simulink model "System_20220515"  (R2020b)
settings: Solver=ode4  StartTime=0.0  StopTime=inf  FixedStep=Ts  RelTol=1e-3  EnableMultiTasking=on
PreLoadFcn:
  | simulation_vars
PostLoadFcn:
  | simulation_vars
InitFcn:
  | simulation_vars
StartFcn:
  | simulation_vars
values from neighbouring files (symbols this model uses):
  ang_variance = 0.001*60    (= 0.06)    [simulation_vars.m]
  bus_va_seed = abs(round(1000*randn(73,1)))    [simulation_vars.m]
  bus_vm_seed = abs(round(1000*randn(73,1)))    [simulation_vars.m]
  event_time_end = event_time_start + 5/60    (= 10000.0833333)    [simulation_vars.m]
  event_time_start = 10000    [simulation_vars.m]
  line_iang0_seed = abs(round(1000*randn(104,1)))    [simulation_vars.m]
  line_iang1_seed = abs(round(1000*randn(104,1)))    [simulation_vars.m]
  line_imag0_seed = abs(round(1000*randn(104,1)))    [simulation_vars.m]
  line_imag1_seed = abs(round(1000*randn(104,1)))    [simulation_vars.m]
  mag_variance = 0.0005    [simulation_vars.m]
  spoof_lower_limit = -pi()/9    [simulation_vars.m]
  spoof_upper_limit = pi()/9    [simulation_vars.m]
  Ts = 0.001    [simulation_vars.m]
  xf_iang0_seed = abs(round(1000*randn(16,1)))    [simulation_vars.m]
  xf_iang1_seed = abs(round(1000*randn(16,1)))    [simulation_vars.m]
  xf_imag0_seed = abs(round(1000*randn(16,1)))    [simulation_vars.m]
  xf_imag1_seed = abs(round(1000*randn(16,1)))    [simulation_vars.m]
undefined symbols (not defined in the file or in its folder): en_spoofing_attack
libraries: rtlab x210, simulink x21, opal_lib x1, rtlab_phasor x1, rtio_spectracom x1
(part 2 of 4)

== system System_20220515/sm_master/PMU202_signals ==
  In1 : Inport
  Demux : Demux  Outputs=8
  PMU202_I1a : rtlab/OpOutput  identifier_use=PMU202_I1a  identifier_hide=PMU202_I1a  nb_parents_identifier=0
      settings: SourceProductName=RT-LAB
  PMU202_I1m : rtlab/OpOutput  identifier_use=PMU202_I1m  identifier_hide=PMU202_I1m  nb_parents_identifier=0
      settings: SourceProductName=RT-LAB
  PMU202_I2a : rtlab/OpOutput  identifier_use=PMU202_I2a  identifier_hide=PMU202_I2a  nb_parents_identifier=0
      settings: SourceProductName=RT-LAB
  PMU202_I2m : rtlab/OpOutput  identifier_use=PMU202_I2m  identifier_hide=PMU202_I2m  nb_parents_identifier=0
      settings: SourceProductName=RT-LAB
  PMU202_I3a : rtlab/OpOutput  identifier_use=PMU202_I3a  identifier_hide=PMU202_I3a  nb_parents_identifier=0
      settings: SourceProductName=RT-LAB
  PMU202_I3m : rtlab/OpOutput  identifier_use=PMU202_I3m  identifier_hide=PMU202_I3m  nb_parents_identifier=0
      settings: SourceProductName=RT-LAB
  PMU202_Va : rtlab/OpOutput  identifier_use=PMU202_Va  identifier_hide=PMU202_Va  nb_parents_identifier=0
      settings: SourceProductName=RT-LAB
  PMU202_Vm : rtlab/OpOutput  identifier_use=PMU202_Vm  identifier_hide=PMU202_Vm  nb_parents_identifier=0
      settings: SourceProductName=RT-LAB
  Spoofing attack : Subsystem
  Out1 : Outport  VectorParamsAs1DForOutWhenUnconnected=off
  wires:
  Demux/3 -> PMU202_I1m/1
  Demux/1 -> PMU202_Vm/1
  Demux/6 -> PMU202_I2a/1
  Demux/2 -> PMU202_Va/1
  Demux/4 -> PMU202_I1a/1
  Demux/5 -> PMU202_I2m/1
  In1/1 -> Spoofing attack/1(Input)
  Demux/7 -> PMU202_I3m/1
  Demux/8 -> PMU202_I3a/1
  Spoofing attack/1(Output) -> Out1/1, Demux/1

== system System_20220515/sm_master/PMU203_signals ==
  In1 : Inport
  Demux : Demux  Outputs=10
  PMU203_I1a : rtlab/OpOutput  identifier_use=PMU203_I1a  identifier_hide=PMU203_I1a  nb_parents_identifier=0
      settings: SourceProductName=RT-LAB
  PMU203_I1m : rtlab/OpOutput  identifier_use=PMU203_I1m  identifier_hide=PMU203_I1m  nb_parents_identifier=0
      settings: SourceProductName=RT-LAB
  PMU203_I2a : rtlab/OpOutput  identifier_use=PMU203_I2a  identifier_hide=PMU203_I2a  nb_parents_identifier=0
      settings: SourceProductName=RT-LAB
  PMU203_I2m : rtlab/OpOutput  identifier_use=PMU203_I2m  identifier_hide=PMU203_I2m  nb_parents_identifier=0
      settings: SourceProductName=RT-LAB
  PMU203_I3a : rtlab/OpOutput  identifier_use=PMU203_I3a  identifier_hide=PMU203_I3a  nb_parents_identifier=0
      settings: SourceProductName=RT-LAB
  PMU203_I3m : rtlab/OpOutput  identifier_use=PMU203_I3m  identifier_hide=PMU203_I3m  nb_parents_identifier=0
      settings: SourceProductName=RT-LAB
  PMU203_I4a : rtlab/OpOutput  identifier_use=PMU203_I4a  identifier_hide=PMU203_I4a  nb_parents_identifier=0
      settings: SourceProductName=RT-LAB
  PMU203_I4m : rtlab/OpOutput  identifier_use=PMU203_I4m  identifier_hide=PMU203_I4m  nb_parents_identifier=0
      settings: SourceProductName=RT-LAB
  PMU203_Va : rtlab/OpOutput  identifier_use=PMU203_Va  identifier_hide=PMU203_Va  nb_parents_identifier=0
      settings: SourceProductName=RT-LAB
  PMU203_Vm : rtlab/OpOutput  identifier_use=PMU203_Vm  identifier_hide=PMU203_Vm  nb_parents_identifier=0
      settings: SourceProductName=RT-LAB
  Spoofing attack : Subsystem
  Out1 : Outport  VectorParamsAs1DForOutWhenUnconnected=off
  wires:
  Demux/10 -> PMU203_I4a/1
  Demux/3 -> PMU203_I1m/1
  Demux/1 -> PMU203_Vm/1
  Demux/6 -> PMU203_I2a/1
  Demux/8 -> PMU203_I3a/1
  Demux/2 -> PMU203_Va/1
  Demux/7 -> PMU203_I3m/1
  Demux/4 -> PMU203_I1a/1
  Demux/5 -> PMU203_I2m/1
  Demux/9 -> PMU203_I4m/1
  In1/1 -> Spoofing attack/1(Input)
  Spoofing attack/1(Output) -> Demux/1, Out1/1

== system System_20220515/sm_master/PMU207_signals ==
  In1 : Inport
  Demux : Demux
  PMU207_I1a : rtlab/OpOutput  identifier_use=PMU207_I1a  identifier_hide=PMU207_I1a  nb_parents_identifier=0
      settings: SourceProductName=RT-LAB
  PMU207_I1m : rtlab/OpOutput  identifier_use=PMU207_I1m  identifier_hide=PMU207_I1m  nb_parents_identifier=0
      settings: SourceProductName=RT-LAB
  PMU207_Va : rtlab/OpOutput  identifier_use=PMU207_Va  identifier_hide=PMU207_Va  nb_parents_identifier=0
      settings: SourceProductName=RT-LAB
  PMU207_Vm : rtlab/OpOutput  identifier_use=PMU207_Vm  identifier_hide=PMU207_Vm  nb_parents_identifier=0
      settings: SourceProductName=RT-LAB
  Spoofing attack : Subsystem
  Out1 : Outport  VectorParamsAs1DForOutWhenUnconnected=off
  wires:
  Demux/1 -> PMU207_Vm/1
  Demux/2 -> PMU207_Va/1
  Demux/4 -> PMU207_I1a/1
  Demux/3 -> PMU207_I1m/1
  In1/1 -> Spoofing attack/1(Input)
  Spoofing attack/1(Output) -> Out1/1, Demux/1

== system System_20220515/sm_master/PMU210_signals ==
  Input : Inport
  Demux : Demux  Outputs=12
  PMU210_I1a : rtlab/OpOutput  identifier_use=PMU210_I1a  identifier_hide=PMU210_I1a  nb_parents_identifier=0
      settings: SourceProductName=RT-LAB
  PMU210_I1m : rtlab/OpOutput  identifier_use=PMU210_I1m  identifier_hide=PMU210_I1m  nb_parents_identifier=0
      settings: SourceProductName=RT-LAB
  PMU210_I2a : rtlab/OpOutput  identifier_use=PMU210_I2a  identifier_hide=PMU210_I2a  nb_parents_identifier=0
      settings: SourceProductName=RT-LAB
  PMU210_I2m : rtlab/OpOutput  identifier_use=PMU210_I2m  identifier_hide=PMU210_I2m  nb_parents_identifier=0
      settings: SourceProductName=RT-LAB
  PMU210_I3a : rtlab/OpOutput  identifier_use=PMU210_I3a  identifier_hide=PMU210_I3a  nb_parents_identifier=0
      settings: SourceProductName=RT-LAB
  PMU210_I3m : rtlab/OpOutput  identifier_use=PMU210_I3m  identifier_hide=PMU210_I3m  nb_parents_identifier=0
      settings: SourceProductName=RT-LAB
  PMU210_I4a : rtlab/OpOutput  identifier_use=PMU210_I4a  identifier_hide=PMU210_I4a  nb_parents_identifier=0
      settings: SourceProductName=RT-LAB
  PMU210_I4m : rtlab/OpOutput  identifier_use=PMU210_I4m  identifier_hide=PMU210_I4m  nb_parents_identifier=0
      settings: SourceProductName=RT-LAB
  PMU210_I5a : rtlab/OpOutput  identifier_use=PMU210_I5a  identifier_hide=PMU210_I5a  nb_parents_identifier=0
      settings: SourceProductName=RT-LAB
  PMU210_I5m : rtlab/OpOutput  identifier_use=PMU210_I5m  identifier_hide=PMU210_I5m  nb_parents_identifier=0
      settings: SourceProductName=RT-LAB
  PMU210_Va : rtlab/OpOutput  identifier_use=PMU210_Va  identifier_hide=PMU210_Va  nb_parents_identifier=0
      settings: SourceProductName=RT-LAB
  PMU210_Vm : rtlab/OpOutput  identifier_use=PMU210_Vm  identifier_hide=PMU210_Vm  nb_parents_identifier=0
      settings: SourceProductName=RT-LAB
  Spoofing attack : Subsystem
  Output : Outport  VectorParamsAs1DForOutWhenUnconnected=off
  wires:
  Demux/1 -> PMU210_Vm/1
  Demux/2 -> PMU210_Va/1
  Demux/3 -> PMU210_I1m/1
  Demux/4 -> PMU210_I1a/1
  Demux/8 -> PMU210_I3a/1
  Demux/9 -> PMU210_I4m/1
  Demux/10 -> PMU210_I4a/1
  Demux/11 -> PMU210_I5m/1
  Demux/12 -> PMU210_I5a/1
  Demux/5 -> PMU210_I2m/1
  Demux/6 -> PMU210_I2a/1
  Demux/7 -> PMU210_I3m/1
  Input/1 -> Spoofing attack/1(Input)
  Spoofing attack/1(Output) -> Output/1, Demux/1

== system System_20220515/sm_master/PMU216_signals ==
  In1 : Inport
  Demux : Demux  Outputs=10
  PMU216_I1a : rtlab/OpOutput  identifier_use=PMU216_I1a  identifier_hide=PMU216_I1a  nb_parents_identifier=0
      settings: SourceProductName=RT-LAB
  PMU216_I1m : rtlab/OpOutput  identifier_use=PMU216_I1m  identifier_hide=PMU216_I1m  nb_parents_identifier=0
      settings: SourceProductName=RT-LAB
  PMU216_I2a : rtlab/OpOutput  identifier_use=PMU216_I2a  identifier_hide=PMU216_I2a  nb_parents_identifier=0
      settings: SourceProductName=RT-LAB
  PMU216_I2m : rtlab/OpOutput  identifier_use=PMU216_I2m  identifier_hide=PMU216_I2m  nb_parents_identifier=0
      settings: SourceProductName=RT-LAB
  PMU216_I3a : rtlab/OpOutput  identifier_use=PMU216_I3a  identifier_hide=PMU216_I3a  nb_parents_identifier=0
      settings: SourceProductName=RT-LAB
  PMU216_I3m : rtlab/OpOutput  identifier_use=PMU216_I3m  identifier_hide=PMU216_I3m  nb_parents_identifier=0
      settings: SourceProductName=RT-LAB
  PMU216_I4a : rtlab/OpOutput  identifier_use=PMU216_I4a  identifier_hide=PMU216_I4a  nb_parents_identifier=0
      settings: SourceProductName=RT-LAB
  PMU216_I4m : rtlab/OpOutput  identifier_use=PMU216_I4m  identifier_hide=PMU216_I4m  nb_parents_identifier=0
      settings: SourceProductName=RT-LAB
  PMU216_Va : rtlab/OpOutput  identifier_use=PMU216_Va  identifier_hide=PMU216_Va  nb_parents_identifier=0
      settings: SourceProductName=RT-LAB
  PMU216_Vm : rtlab/OpOutput  identifier_use=PMU216_Vm  identifier_hide=PMU216_Vm  nb_parents_identifier=0
      settings: SourceProductName=RT-LAB
  Spoofing attack : Subsystem
  Out1 : Outport  VectorParamsAs1DForOutWhenUnconnected=off
  wires:
  Demux/10 -> PMU216_I4a/1
  Demux/3 -> PMU216_I1m/1
  Demux/1 -> PMU216_Vm/1
  Demux/6 -> PMU216_I2a/1
  Demux/8 -> PMU216_I3a/1
  Demux/2 -> PMU216_Va/1
  Demux/7 -> PMU216_I3m/1
  Demux/4 -> PMU216_I1a/1
  Demux/5 -> PMU216_I2m/1
  Demux/9 -> PMU216_I4m/1
  In1/1 -> Spoofing attack/1(Input)
  Spoofing attack/1(Output) -> Demux/1, Out1/1

== system System_20220515/sm_master/PMU221_signals ==
  In1 : Inport
  Demux : Demux  Outputs=12
  PMU221_I1a : rtlab/OpOutput  identifier_use=PMU221_I1a  identifier_hide=PMU221_I1a  nb_parents_identifier=0
      settings: SourceProductName=RT-LAB
  PMU221_I1m : rtlab/OpOutput  identifier_use=PMU221_I1m  identifier_hide=PMU221_I1m  nb_parents_identifier=0
      settings: SourceProductName=RT-LAB
  PMU221_I2a : rtlab/OpOutput  identifier_use=PMU221_I2a  identifier_hide=PMU221_I2a  nb_parents_identifier=0
      settings: SourceProductName=RT-LAB
  PMU221_I2m : rtlab/OpOutput  identifier_use=PMU221_I2m  identifier_hide=PMU221_I2m  nb_parents_identifier=0
      settings: SourceProductName=RT-LAB
  PMU221_I3a : rtlab/OpOutput  identifier_use=PMU221_I3a  identifier_hide=PMU221_I3a  nb_parents_identifier=0
      settings: SourceProductName=RT-LAB
  PMU221_I3m : rtlab/OpOutput  identifier_use=PMU221_I3m  identifier_hide=PMU221_I3m  nb_parents_identifier=0
      settings: SourceProductName=RT-LAB
  PMU221_I4a : rtlab/OpOutput  identifier_use=PMU221_I4a  identifier_hide=PMU221_I4a  nb_parents_identifier=0
      settings: SourceProductName=RT-LAB
  PMU221_I4m : rtlab/OpOutput  identifier_use=PMU221_I4m  identifier_hide=PMU221_I4m  nb_parents_identifier=0
      settings: SourceProductName=RT-LAB
  PMU221_I5a : rtlab/OpOutput  identifier_use=PMU221_I5a  identifier_hide=PMU221_I5a  nb_parents_identifier=0
      settings: SourceProductName=RT-LAB
  PMU221_I5m : rtlab/OpOutput  identifier_use=PMU221_I5m  identifier_hide=PMU221_I5m  nb_parents_identifier=0
      settings: SourceProductName=RT-LAB
  PMU221_Va : rtlab/OpOutput  identifier_use=PMU221_Va  identifier_hide=PMU221_Va  nb_parents_identifier=0
      settings: SourceProductName=RT-LAB
  PMU221_Vm : rtlab/OpOutput  identifier_use=PMU221_Vm  identifier_hide=PMU221_Vm  nb_parents_identifier=0
      settings: SourceProductName=RT-LAB
  Spoofing attack : Subsystem
  Out1 : Outport  VectorParamsAs1DForOutWhenUnconnected=off
  wires:
  Demux/1 -> PMU221_Vm/1
  Demux/2 -> PMU221_Va/1
  Demux/3 -> PMU221_I1m/1
  Demux/4 -> PMU221_I1a/1
  Demux/8 -> PMU221_I3a/1
  Demux/9 -> PMU221_I4m/1
  Demux/10 -> PMU221_I4a/1
  Demux/11 -> PMU221_I5m/1
  Demux/12 -> PMU221_I5a/1
  Demux/5 -> PMU221_I2m/1
  Demux/6 -> PMU221_I2a/1
  Demux/7 -> PMU221_I3m/1
  In1/1 -> Spoofing attack/1(Input)
  Spoofing attack/1(Output) -> Out1/1, Demux/1

== system System_20220515/sm_master/PMU223_signals ==
  Input : Inport
  Demux : Demux  Outputs=12
  PMU223_I1a : rtlab/OpOutput  identifier_use=PMU223_I1a  identifier_hide=PMU223_I1a  nb_parents_identifier=0
      settings: SourceProductName=RT-LAB
  PMU223_I1m : rtlab/OpOutput  identifier_use=PMU223_I1m  identifier_hide=PMU223_I1m  nb_parents_identifier=0
      settings: SourceProductName=RT-LAB
  PMU223_I2a : rtlab/OpOutput  identifier_use=PMU223_I2a  identifier_hide=PMU223_I2a  nb_parents_identifier=0
      settings: SourceProductName=RT-LAB
  PMU223_I2m : rtlab/OpOutput  identifier_use=PMU223_I2m  identifier_hide=PMU223_I2m  nb_parents_identifier=0
      settings: SourceProductName=RT-LAB
  PMU223_I3a : rtlab/OpOutput  identifier_use=PMU223_I3a  identifier_hide=PMU223_I3a  nb_parents_identifier=0
      settings: SourceProductName=RT-LAB
  PMU223_I3m : rtlab/OpOutput  identifier_use=PMU223_I3m  identifier_hide=PMU223_I3m  nb_parents_identifier=0
      settings: SourceProductName=RT-LAB
  PMU223_I4a : rtlab/OpOutput  identifier_use=PMU223_I4a  identifier_hide=PMU223_I4a  nb_parents_identifier=0
      settings: SourceProductName=RT-LAB
  PMU223_I4m : rtlab/OpOutput  identifier_use=PMU223_I4m  identifier_hide=PMU223_I4m  nb_parents_identifier=0
      settings: SourceProductName=RT-LAB
  PMU223_I5a : rtlab/OpOutput  identifier_use=PMU223_I5a  identifier_hide=PMU223_I5a  nb_parents_identifier=0
      settings: SourceProductName=RT-LAB
  PMU223_I5m : rtlab/OpOutput  identifier_use=PMU223_I5m  identifier_hide=PMU223_I5m  nb_parents_identifier=0
      settings: SourceProductName=RT-LAB
  PMU223_Va : rtlab/OpOutput  identifier_use=PMU223_Va  identifier_hide=PMU223_Va  nb_parents_identifier=0
      settings: SourceProductName=RT-LAB
  PMU223_Vm : rtlab/OpOutput  identifier_use=PMU223_Vm  identifier_hide=PMU223_Vm  nb_parents_identifier=0
      settings: SourceProductName=RT-LAB
  Spoofing attack : Subsystem
  Output : Outport  VectorParamsAs1DForOutWhenUnconnected=off
  wires:
  Demux/1 -> PMU223_Vm/1
  Demux/2 -> PMU223_Va/1
  Demux/3 -> PMU223_I1m/1
  Demux/4 -> PMU223_I1a/1
  Demux/8 -> PMU223_I3a/1
  Demux/9 -> PMU223_I4m/1
  Demux/10 -> PMU223_I4a/1
  Demux/11 -> PMU223_I5m/1
  Demux/12 -> PMU223_I5a/1
  Demux/5 -> PMU223_I2m/1
  Demux/6 -> PMU223_I2a/1
  Demux/7 -> PMU223_I3m/1
  Input/1 -> Spoofing attack/1(Input)
  Spoofing attack/1(Output) -> Output/1, Demux/1

== system System_20220515/sm_master/PMU302_signals ==
  In1 : Inport
  Demux : Demux  Outputs=8
  PMU302_I1a : rtlab/OpOutput  identifier_use=PMU302_I1a  identifier_hide=PMU302_I1a  nb_parents_identifier=0
      settings: SourceProductName=RT-LAB
  PMU302_I1m : rtlab/OpOutput  identifier_use=PMU302_I1m  identifier_hide=PMU302_I1m  nb_parents_identifier=0
      settings: SourceProductName=RT-LAB
  PMU302_I2a : rtlab/OpOutput  identifier_use=PMU302_I2a  identifier_hide=PMU302_I2a  nb_parents_identifier=0
      settings: SourceProductName=RT-LAB
  PMU302_I2m : rtlab/OpOutput  identifier_use=PMU302_I2m  identifier_hide=PMU302_I2m  nb_parents_identifier=0
      settings: SourceProductName=RT-LAB
  PMU302_I3a : rtlab/OpOutput  identifier_use=PMU302_I3a  identifier_hide=PMU302_I3a  nb_parents_identifier=0
      settings: SourceProductName=RT-LAB
  PMU302_I3m : rtlab/OpOutput  identifier_use=PMU302_I3m  identifier_hide=PMU302_I3m  nb_parents_identifier=0
      settings: SourceProductName=RT-LAB
  PMU302_Va : rtlab/OpOutput  identifier_use=PMU302_Va  identifier_hide=PMU302_Va  nb_parents_identifier=0
      settings: SourceProductName=RT-LAB
  PMU302_Vm : rtlab/OpOutput  identifier_use=PMU302_Vm  identifier_hide=PMU302_Vm  nb_parents_identifier=0
      settings: SourceProductName=RT-LAB
  Spoofing attack : Subsystem
  Out1 : Outport  VectorParamsAs1DForOutWhenUnconnected=off
  wires:
  In1/1 -> Spoofing attack/1(Input)
  Demux/2 -> PMU302_Va/1
  Demux/1 -> PMU302_Vm/1
  Demux/3 -> PMU302_I1m/1
  Demux/4 -> PMU302_I1a/1
  Demux/5 -> PMU302_I2m/1
  Demux/6 -> PMU302_I2a/1
  Demux/7 -> PMU302_I3m/1
  Demux/8 -> PMU302_I3a/1
  Spoofing attack/1(Output) -> Out1/1, Demux/1

== system System_20220515/sm_master/PMU303_signals ==
  In1 : Inport
  Demux : Demux  Outputs=8
  PMU303_I1a : rtlab/OpOutput  identifier_use=PMU303_I1a  identifier_hide=PMU303_I1a  nb_parents_identifier=0
      settings: SourceProductName=RT-LAB
  PMU303_I1m : rtlab/OpOutput  identifier_use=PMU303_I1m  identifier_hide=PMU303_I1m  nb_parents_identifier=0
      settings: SourceProductName=RT-LAB
  PMU303_I2a : rtlab/OpOutput  identifier_use=PMU303_I2a  identifier_hide=PMU303_I2a  nb_parents_identifier=0
      settings: SourceProductName=RT-LAB
  PMU303_I2m : rtlab/OpOutput  identifier_use=PMU303_I2m  identifier_hide=PMU303_I2m  nb_parents_identifier=0
      settings: SourceProductName=RT-LAB
  PMU303_I3a : rtlab/OpOutput  identifier_use=PMU303_I3a  identifier_hide=PMU303_I3a  nb_parents_identifier=0
      settings: SourceProductName=RT-LAB
  PMU303_I3m : rtlab/OpOutput  identifier_use=PMU303_I3m  identifier_hide=PMU303_I3m  nb_parents_identifier=0
      settings: SourceProductName=RT-LAB
  PMU303_Va : rtlab/OpOutput  identifier_use=PMU303_Va  identifier_hide=PMU303_Va  nb_parents_identifier=0
      settings: SourceProductName=RT-LAB
  PMU303_Vm : rtlab/OpOutput  identifier_use=PMU303_Vm  identifier_hide=PMU303_Vm  nb_parents_identifier=0
      settings: SourceProductName=RT-LAB
  Spoofing attack : Subsystem
  Out1 : Outport  VectorParamsAs1DForOutWhenUnconnected=off
  wires:
  In1/1 -> Spoofing attack/1(Input)
  Demux/1 -> PMU303_Vm/1
  Demux/2 -> PMU303_Va/1
  Demux/3 -> PMU303_I1m/1
  Demux/4 -> PMU303_I1a/1
  Demux/5 -> PMU303_I2m/1
  Demux/6 -> PMU303_I2a/1
  Demux/7 -> PMU303_I3m/1
  Demux/8 -> PMU303_I3a/1
  Spoofing attack/1(Output) -> Out1/1, Demux/1

== system System_20220515/sm_master/PMU307_signals ==
  In1 : Inport
  Demux : Demux
  PMU307_I1a : rtlab/OpOutput  identifier_use=PMU307_I1a  identifier_hide=PMU307_I1a  nb_parents_identifier=0
      settings: SourceProductName=RT-LAB
  PMU307_I1m : rtlab/OpOutput  identifier_use=PMU307_I1m  identifier_hide=PMU307_I1m  nb_parents_identifier=0
      settings: SourceProductName=RT-LAB
  PMU307_Va : rtlab/OpOutput  identifier_use=PMU307_Va  identifier_hide=PMU307_Va  nb_parents_identifier=0
      settings: SourceProductName=RT-LAB
  PMU307_Vm : rtlab/OpOutput  identifier_use=PMU307_Vm  identifier_hide=PMU307_Vm  nb_parents_identifier=0
      settings: SourceProductName=RT-LAB
  Spoofing attack : Subsystem
  Out1 : Outport  VectorParamsAs1DForOutWhenUnconnected=off
  wires:
  In1/1 -> Spoofing attack/1(Input)
  Demux/1 -> PMU307_Vm/1
  Demux/2 -> PMU307_Va/1
  Demux/4 -> PMU307_I1a/1
  Demux/3 -> PMU307_I1m/1
  Spoofing attack/1(Output) -> Demux/1, Out1/1

== system System_20220515/sm_master/PMU310_signals ==
  In1 : Inport
  Demux : Demux  Outputs=12
  PMU310_I1a : rtlab/OpOutput  identifier_use=PMU310_I1a  identifier_hide=PMU310_I1a  nb_parents_identifier=0
      settings: SourceProductName=RT-LAB
  PMU310_I1m : rtlab/OpOutput  identifier_use=PMU310_I1m  identifier_hide=PMU310_I1m  nb_parents_identifier=0
      settings: SourceProductName=RT-LAB
  PMU310_I2a : rtlab/OpOutput  identifier_use=PMU310_I2a  identifier_hide=PMU310_I2a  nb_parents_identifier=0
      settings: SourceProductName=RT-LAB
  PMU310_I2m : rtlab/OpOutput  identifier_use=PMU310_I2m  identifier_hide=PMU310_I2m  nb_parents_identifier=0
      settings: SourceProductName=RT-LAB
  PMU310_I3a : rtlab/OpOutput  identifier_use=PMU310_I3a  identifier_hide=PMU310_I3a  nb_parents_identifier=0
      settings: SourceProductName=RT-LAB
  PMU310_I3m : rtlab/OpOutput  identifier_use=PMU310_I3m  identifier_hide=PMU310_I3m  nb_parents_identifier=0
      settings: SourceProductName=RT-LAB
  PMU310_I4a : rtlab/OpOutput  identifier_use=PMU310_I4a  identifier_hide=PMU310_I4a  nb_parents_identifier=0
      settings: SourceProductName=RT-LAB
  PMU310_I4m : rtlab/OpOutput  identifier_use=PMU310_I4m  identifier_hide=PMU310_I4m  nb_parents_identifier=0
      settings: SourceProductName=RT-LAB
  PMU310_I5a : rtlab/OpOutput  identifier_use=PMU310_I5a  identifier_hide=PMU310_I5a  nb_parents_identifier=0
      settings: SourceProductName=RT-LAB
  PMU310_I5m : rtlab/OpOutput  identifier_use=PMU310_I5m  identifier_hide=PMU310_I5m  nb_parents_identifier=0
      settings: SourceProductName=RT-LAB
  PMU310_Va : rtlab/OpOutput  identifier_use=PMU310_Va  identifier_hide=PMU310_Va  nb_parents_identifier=0
      settings: SourceProductName=RT-LAB
  PMU310_Vm : rtlab/OpOutput  identifier_use=PMU310_Vm  identifier_hide=PMU310_Vm  nb_parents_identifier=0
      settings: SourceProductName=RT-LAB
  Spoofing attack : Subsystem
  Out1 : Outport  VectorParamsAs1DForOutWhenUnconnected=off
  wires:
  In1/1 -> Spoofing attack/1(Input)
  Demux/1 -> PMU310_Vm/1
  Demux/2 -> PMU310_Va/1
  Demux/3 -> PMU310_I1m/1
  Demux/4 -> PMU310_I1a/1
  Demux/5 -> PMU310_I2m/1
  Demux/6 -> PMU310_I2a/1
  Demux/7 -> PMU310_I3m/1
  Demux/8 -> PMU310_I3a/1
  Demux/9 -> PMU310_I4m/1
  Demux/10 -> PMU310_I4a/1
  Demux/11 -> PMU310_I5m/1
  Demux/12 -> PMU310_I5a/1
  Spoofing attack/1(Output) -> Out1/1, Demux/1

== system System_20220515/sm_master/PMU316_signals ==
  In1 : Inport
  Demux : Demux  Outputs=10
  PMU316_I1a : rtlab/OpOutput  identifier_use=PMU316_I1a  identifier_hide=PMU316_I1a  nb_parents_identifier=0
      settings: SourceProductName=RT-LAB
  PMU316_I1m : rtlab/OpOutput  identifier_use=PMU316_I1m  identifier_hide=PMU316_I1m  nb_parents_identifier=0
      settings: SourceProductName=RT-LAB
  PMU316_I2a : rtlab/OpOutput  identifier_use=PMU316_I2a  identifier_hide=PMU316_I2a  nb_parents_identifier=0
      settings: SourceProductName=RT-LAB
  PMU316_I2m : rtlab/OpOutput  identifier_use=PMU316_I2m  identifier_hide=PMU316_I2m  nb_parents_identifier=0
      settings: SourceProductName=RT-LAB
  PMU316_I3a : rtlab/OpOutput  identifier_use=PMU316_I3a  identifier_hide=PMU316_I3a  nb_parents_identifier=0
      settings: SourceProductName=RT-LAB
  PMU316_I3m : rtlab/OpOutput  identifier_use=PMU316_I3m  identifier_hide=PMU316_I3m  nb_parents_identifier=0
      settings: SourceProductName=RT-LAB
  PMU316_I4a : rtlab/OpOutput  identifier_use=PMU316_I4a  identifier_hide=PMU316_I4a  nb_parents_identifier=0
      settings: SourceProductName=RT-LAB
  PMU316_I4m : rtlab/OpOutput  identifier_use=PMU316_I4m  identifier_hide=PMU316_I4m  nb_parents_identifier=0
      settings: SourceProductName=RT-LAB
  PMU316_Va : rtlab/OpOutput  identifier_use=PMU316_Va  identifier_hide=PMU316_Va  nb_parents_identifier=0
      settings: SourceProductName=RT-LAB
  PMU316_Vm : rtlab/OpOutput  identifier_use=PMU316_Vm  identifier_hide=PMU316_Vm  nb_parents_identifier=0
      settings: SourceProductName=RT-LAB
  Spoofing attack : Subsystem
  Out1 : Outport  VectorParamsAs1DForOutWhenUnconnected=off
  wires:
  Demux/10 -> PMU316_I4a/1
  Demux/3 -> PMU316_I1m/1
  Demux/1 -> PMU316_Vm/1
  Demux/6 -> PMU316_I2a/1
  Demux/8 -> PMU316_I3a/1
  Demux/2 -> PMU316_Va/1
  Demux/7 -> PMU316_I3m/1
  Demux/4 -> PMU316_I1a/1
  Demux/5 -> PMU316_I2m/1
  Demux/9 -> PMU316_I4m/1
  In1/1 -> Spoofing attack/1(Input)
  Spoofing attack/1(Output) -> Demux/1, Out1/1

== system System_20220515/sm_master/PMU321_signals ==
  In1 : Inport
  Demux : Demux  Outputs=12
  PMU321_I1a : rtlab/OpOutput  identifier_use=PMU321_I1a  identifier_hide=PMU321_I1a  nb_parents_identifier=0
      settings: SourceProductName=RT-LAB
  PMU321_I1m : rtlab/OpOutput  identifier_use=PMU321_I1m  identifier_hide=PMU321_I1m  nb_parents_identifier=0
      settings: SourceProductName=RT-LAB
  PMU321_I2a : rtlab/OpOutput  identifier_use=PMU321_I2a  identifier_hide=PMU321_I2a  nb_parents_identifier=0
      settings: SourceProductName=RT-LAB
  PMU321_I2m : rtlab/OpOutput  identifier_use=PMU321_I2m  identifier_hide=PMU321_I2m  nb_parents_identifier=0
      settings: SourceProductName=RT-LAB
  PMU321_I3a : rtlab/OpOutput  identifier_use=PMU321_I3a  identifier_hide=PMU321_I3a  nb_parents_identifier=0
      settings: SourceProductName=RT-LAB
  PMU321_I3m : rtlab/OpOutput  identifier_use=PMU321_I3m  identifier_hide=PMU321_I3m  nb_parents_identifier=0
      settings: SourceProductName=RT-LAB
  PMU321_I4a : rtlab/OpOutput  identifier_use=PMU321_I4a  identifier_hide=PMU321_I4a  nb_parents_identifier=0
      settings: SourceProductName=RT-LAB
  PMU321_I4m : rtlab/OpOutput  identifier_use=PMU321_I4m  identifier_hide=PMU321_I4m  nb_parents_identifier=0
      settings: SourceProductName=RT-LAB
  PMU321_I5a : rtlab/OpOutput  identifier_use=PMU321_I5a  identifier_hide=PMU321_I5a  nb_parents_identifier=0
      settings: SourceProductName=RT-LAB
  PMU321_I5m : rtlab/OpOutput  identifier_use=PMU321_I5m  identifier_hide=PMU321_I5m  nb_parents_identifier=0
      settings: SourceProductName=RT-LAB
  PMU321_Va : rtlab/OpOutput  identifier_use=PMU321_Va  identifier_hide=PMU321_Va  nb_parents_identifier=0
      settings: SourceProductName=RT-LAB
  PMU321_Vm : rtlab/OpOutput  identifier_use=PMU321_Vm  identifier_hide=PMU321_Vm  nb_parents_identifier=0
      settings: SourceProductName=RT-LAB
  Spoofing attack : Subsystem
  Out1 : Outport  VectorParamsAs1DForOutWhenUnconnected=off
  wires:
  In1/1 -> Spoofing attack/1(Input)
  Spoofing attack/1(Output) -> Out1/1, Demux/1
  Demux/1 -> PMU321_Vm/1
  Demux/2 -> PMU321_Va/1
  Demux/3 -> PMU321_I1m/1
  Demux/4 -> PMU321_I1a/1
  Demux/5 -> PMU321_I2m/1
  Demux/6 -> PMU321_I2a/1
  Demux/7 -> PMU321_I3m/1
  Demux/8 -> PMU321_I3a/1
  Demux/9 -> PMU321_I4m/1
  Demux/10 -> PMU321_I4a/1
  Demux/11 -> PMU321_I5m/1
  Demux/12 -> PMU321_I5a/1

== system System_20220515/sm_master/PMU323_signals ==
  In1 : Inport
  Demux : Demux  Outputs=12
  PMU323_I1a : rtlab/OpOutput  identifier_use=PMU323_I1a  identifier_hide=PMU323_I1a  nb_parents_identifier=0
      settings: SourceProductName=RT-LAB
  PMU323_I1m : rtlab/OpOutput  identifier_use=PMU323_I1m  identifier_hide=PMU323_I1m  nb_parents_identifier=0
      settings: SourceProductName=RT-LAB
  PMU323_I2a : rtlab/OpOutput  identifier_use=PMU323_I2a  identifier_hide=PMU323_I2a  nb_parents_identifier=0
      settings: SourceProductName=RT-LAB
  PMU323_I2m : rtlab/OpOutput  identifier_use=PMU323_I2m  identifier_hide=PMU323_I2m  nb_parents_identifier=0
      settings: SourceProductName=RT-LAB
  PMU323_I3a : rtlab/OpOutput  identifier_use=PMU323_I3a  identifier_hide=PMU323_I3a  nb_parents_identifier=0
      settings: SourceProductName=RT-LAB
  PMU323_I3m : rtlab/OpOutput  identifier_use=PMU323_I3m  identifier_hide=PMU323_I3m  nb_parents_identifier=0
      settings: SourceProductName=RT-LAB
  PMU323_I4a : rtlab/OpOutput  identifier_use=PMU323_I4a  identifier_hide=PMU323_I4a  nb_parents_identifier=0
      settings: SourceProductName=RT-LAB
  PMU323_I4m : rtlab/OpOutput  identifier_use=PMU323_I4m  identifier_hide=PMU323_I4m  nb_parents_identifier=0
      settings: SourceProductName=RT-LAB
  PMU323_I5a : rtlab/OpOutput  identifier_use=PMU323_I5a  identifier_hide=PMU323_I5a  nb_parents_identifier=0
      settings: SourceProductName=RT-LAB
  PMU323_I5m : rtlab/OpOutput  identifier_use=PMU323_I5m  identifier_hide=PMU323_I5m  nb_parents_identifier=0
      settings: SourceProductName=RT-LAB
  PMU323_Va : rtlab/OpOutput  identifier_use=PMU323_Va  identifier_hide=PMU323_Va  nb_parents_identifier=0
      settings: SourceProductName=RT-LAB
  PMU323_Vm : rtlab/OpOutput  identifier_use=PMU323_Vm  identifier_hide=PMU323_Vm  nb_parents_identifier=0
      settings: SourceProductName=RT-LAB
  Spoofing attack : Subsystem
  Out1 : Outport  VectorParamsAs1DForOutWhenUnconnected=off
  wires:
  In1/1 -> Spoofing attack/1(Input)
  Spoofing attack/1(Output) -> Demux/1, Out1/1
  Demux/1 -> PMU323_Vm/1
  Demux/2 -> PMU323_Va/1
  Demux/3 -> PMU323_I1m/1
  Demux/4 -> PMU323_I1a/1
  Demux/5 -> PMU323_I2m/1
  Demux/6 -> PMU323_I2a/1
  Demux/7 -> PMU323_I3m/1
  Demux/8 -> PMU323_I3a/1
  Demux/9 -> PMU323_I4m/1
  Demux/10 -> PMU323_I4a/1
  Demux/11 -> PMU323_I5m/1
  Demux/12 -> PMU323_I5a/1

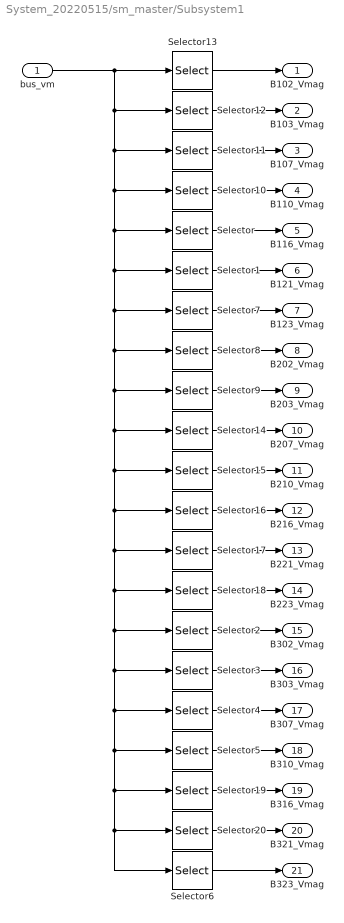
== system System_20220515/sm_master/Subsystem1 ==
  bus_vm : Inport
  Selector : Selector  InputPortWidth=73  IndexOptions=Index vector (dialog)  Indices=16  OutputSizes=1
  Selector1 : Selector  InputPortWidth=73  IndexOptions=Index vector (dialog)  Indices=21  OutputSizes=1
  Selector10 : Selector  InputPortWidth=73  IndexOptions=Index vector (dialog)  Indices=10  OutputSizes=1
  Selector11 : Selector  InputPortWidth=73  IndexOptions=Index vector (dialog)  Indices=7  OutputSizes=1
  Selector12 : Selector  InputPortWidth=73  IndexOptions=Index vector (dialog)  Indices=3  OutputSizes=1
  Selector13 : Selector  InputPortWidth=73  IndexOptions=Index vector (dialog)  Indices=2  OutputSizes=1
  Selector14 : Selector  InputPortWidth=73  IndexOptions=Index vector (dialog)  Indices=31  OutputSizes=1
  Selector15 : Selector  InputPortWidth=73  IndexOptions=Index vector (dialog)  Indices=34  OutputSizes=1
  Selector16 : Selector  InputPortWidth=73  IndexOptions=Index vector (dialog)  Indices=40  OutputSizes=1
  Selector17 : Selector  InputPortWidth=73  IndexOptions=Index vector (dialog)  Indices=45  OutputSizes=1
  Selector18 : Selector  InputPortWidth=73  IndexOptions=Index vector (dialog)  Indices=47  OutputSizes=1
  Selector19 : Selector  InputPortWidth=73  IndexOptions=Index vector (dialog)  Indices=64  OutputSizes=1
  Selector2 : Selector  InputPortWidth=73  IndexOptions=Index vector (dialog)  Indices=50  OutputSizes=1
  Selector20 : Selector  InputPortWidth=73  IndexOptions=Index vector (dialog)  Indices=69  OutputSizes=1
  Selector3 : Selector  InputPortWidth=73  IndexOptions=Index vector (dialog)  Indices=51  OutputSizes=1
  Selector4 : Selector  InputPortWidth=73  IndexOptions=Index vector (dialog)  Indices=55  OutputSizes=1
  Selector5 : Selector  InputPortWidth=73  IndexOptions=Index vector (dialog)  Indices=58  OutputSizes=1
  Selector6 : Selector  InputPortWidth=73  IndexOptions=Index vector (dialog)  Indices=71  OutputSizes=1
  Selector7 : Selector  InputPortWidth=73  IndexOptions=Index vector (dialog)  Indices=23  OutputSizes=1
  Selector8 : Selector  InputPortWidth=73  IndexOptions=Index vector (dialog)  Indices=26  OutputSizes=1
  Selector9 : Selector  InputPortWidth=73  IndexOptions=Index vector (dialog)  Indices=27  OutputSizes=1
  B102_Vmag : Outport  VectorParamsAs1DForOutWhenUnconnected=off
  B103_Vmag : Outport  Port=2  VectorParamsAs1DForOutWhenUnconnected=off
  B107_Vmag : Outport  Port=3  VectorParamsAs1DForOutWhenUnconnected=off
  B110_Vmag : Outport  Port=4  VectorParamsAs1DForOutWhenUnconnected=off
  B116_Vmag : Outport  Port=5  VectorParamsAs1DForOutWhenUnconnected=off
  B121_Vmag : Outport  Port=6  VectorParamsAs1DForOutWhenUnconnected=off
  B123_Vmag : Outport  Port=7  VectorParamsAs1DForOutWhenUnconnected=off
  B202_Vmag : Outport  Port=8  VectorParamsAs1DForOutWhenUnconnected=off
  B203_Vmag : Outport  Port=9  VectorParamsAs1DForOutWhenUnconnected=off
  B207_Vmag : Outport  Port=10  VectorParamsAs1DForOutWhenUnconnected=off
  B210_Vmag : Outport  Port=11  VectorParamsAs1DForOutWhenUnconnected=off
  B216_Vmag : Outport  Port=12  VectorParamsAs1DForOutWhenUnconnected=off
  B221_Vmag : Outport  Port=13  VectorParamsAs1DForOutWhenUnconnected=off
  B223_Vmag : Outport  Port=14  VectorParamsAs1DForOutWhenUnconnected=off
  B302_Vmag : Outport  Port=15  VectorParamsAs1DForOutWhenUnconnected=off
  B303_Vmag : Outport  Port=16  VectorParamsAs1DForOutWhenUnconnected=off
  B307_Vmag : Outport  Port=17  VectorParamsAs1DForOutWhenUnconnected=off
  B310_Vmag : Outport  Port=18  VectorParamsAs1DForOutWhenUnconnected=off
  B316_Vmag : Outport  Port=19  VectorParamsAs1DForOutWhenUnconnected=off
  B321_Vmag : Outport  Port=20  VectorParamsAs1DForOutWhenUnconnected=off
  B323_Vmag : Outport  Port=21  VectorParamsAs1DForOutWhenUnconnected=off
  wires:
  Selector/1 -> B116_Vmag/1
  Selector1/1 -> B121_Vmag/1
  Selector2/1 -> B302_Vmag/1
  Selector3/1 -> B303_Vmag/1
  Selector4/1 -> B307_Vmag/1
  Selector5/1 -> B310_Vmag/1
  Selector6/1 -> B323_Vmag/1
  Selector10/1 -> B110_Vmag/1
  Selector11/1 -> B107_Vmag/1
  Selector12/1 -> B103_Vmag/1
  Selector13/1 -> B102_Vmag/1
  Selector7/1 -> B123_Vmag/1
  Selector8/1 -> B202_Vmag/1
  Selector9/1 -> B203_Vmag/1
  Selector14/1 -> B207_Vmag/1
  Selector15/1 -> B210_Vmag/1
  Selector16/1 -> B216_Vmag/1
  Selector17/1 -> B221_Vmag/1
  Selector18/1 -> B223_Vmag/1
  Selector19/1 -> B316_Vmag/1
  Selector20/1 -> B321_Vmag/1
  bus_vm/1 -> Selector6/1, Selector20/1, Selector19/1, Selector5/1, Selector4/1, Selector3/1, Selector2/1, Selector18/1, Selector17/1, Selector16/1, Selector15/1, Selector14/1, Selector9/1, Selector8/1, Selector7/1, Selector1/1, Selector/1, Selector10/1, Selector11/1, Selector12/1, Selector13/1

== system System_20220515/sm_master/Subsystem10 ==
  note: Iang1
  Iang1 : Inport
  Terminator : Terminator
  wires:
  Iang1/1 -> Terminator/1

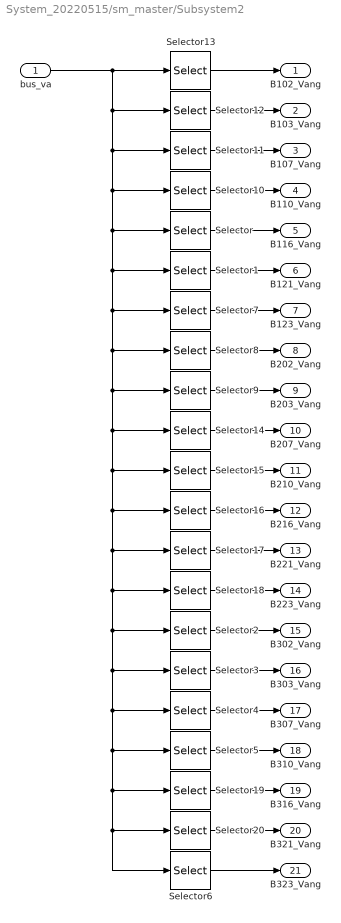
== system System_20220515/sm_master/Subsystem2 ==
  bus_va : Inport
  Selector : Selector  InputPortWidth=73  IndexOptions=Index vector (dialog)  Indices=16  OutputSizes=1
  Selector1 : Selector  InputPortWidth=73  IndexOptions=Index vector (dialog)  Indices=21  OutputSizes=1
  Selector10 : Selector  InputPortWidth=73  IndexOptions=Index vector (dialog)  Indices=10  OutputSizes=1
  Selector11 : Selector  InputPortWidth=73  IndexOptions=Index vector (dialog)  Indices=7  OutputSizes=1
  Selector12 : Selector  InputPortWidth=73  IndexOptions=Index vector (dialog)  Indices=3  OutputSizes=1
  Selector13 : Selector  InputPortWidth=73  IndexOptions=Index vector (dialog)  Indices=2  OutputSizes=1
  Selector14 : Selector  InputPortWidth=73  IndexOptions=Index vector (dialog)  Indices=31  OutputSizes=1
  Selector15 : Selector  InputPortWidth=73  IndexOptions=Index vector (dialog)  Indices=34  OutputSizes=1
  Selector16 : Selector  InputPortWidth=73  IndexOptions=Index vector (dialog)  Indices=40  OutputSizes=1
  Selector17 : Selector  InputPortWidth=73  IndexOptions=Index vector (dialog)  Indices=45  OutputSizes=1
  Selector18 : Selector  InputPortWidth=73  IndexOptions=Index vector (dialog)  Indices=47  OutputSizes=1
  Selector19 : Selector  InputPortWidth=73  IndexOptions=Index vector (dialog)  Indices=64  OutputSizes=1
  Selector2 : Selector  InputPortWidth=73  IndexOptions=Index vector (dialog)  Indices=50  OutputSizes=1
  Selector20 : Selector  InputPortWidth=73  IndexOptions=Index vector (dialog)  Indices=69  OutputSizes=1
  Selector3 : Selector  InputPortWidth=73  IndexOptions=Index vector (dialog)  Indices=51  OutputSizes=1
  Selector4 : Selector  InputPortWidth=73  IndexOptions=Index vector (dialog)  Indices=55  OutputSizes=1
  Selector5 : Selector  InputPortWidth=73  IndexOptions=Index vector (dialog)  Indices=58  OutputSizes=1
  Selector6 : Selector  InputPortWidth=73  IndexOptions=Index vector (dialog)  Indices=71  OutputSizes=1
  Selector7 : Selector  InputPortWidth=73  IndexOptions=Index vector (dialog)  Indices=23  OutputSizes=1
  Selector8 : Selector  InputPortWidth=73  IndexOptions=Index vector (dialog)  Indices=26  OutputSizes=1
  Selector9 : Selector  InputPortWidth=73  IndexOptions=Index vector (dialog)  Indices=27  OutputSizes=1
  B102_Vang : Outport  VectorParamsAs1DForOutWhenUnconnected=off
  B103_Vang : Outport  Port=2  VectorParamsAs1DForOutWhenUnconnected=off
  B107_Vang : Outport  Port=3  VectorParamsAs1DForOutWhenUnconnected=off
  B110_Vang : Outport  Port=4  VectorParamsAs1DForOutWhenUnconnected=off
  B116_Vang : Outport  Port=5  VectorParamsAs1DForOutWhenUnconnected=off
  B121_Vang : Outport  Port=6  VectorParamsAs1DForOutWhenUnconnected=off
  B123_Vang : Outport  Port=7  VectorParamsAs1DForOutWhenUnconnected=off
  B202_Vang : Outport  Port=8  VectorParamsAs1DForOutWhenUnconnected=off
  B203_Vang : Outport  Port=9  VectorParamsAs1DForOutWhenUnconnected=off
  B207_Vang : Outport  Port=10  VectorParamsAs1DForOutWhenUnconnected=off
  B210_Vang : Outport  Port=11  VectorParamsAs1DForOutWhenUnconnected=off
  B216_Vang : Outport  Port=12  VectorParamsAs1DForOutWhenUnconnected=off
  B221_Vang : Outport  Port=13  VectorParamsAs1DForOutWhenUnconnected=off
  B223_Vang : Outport  Port=14  VectorParamsAs1DForOutWhenUnconnected=off
  B302_Vang : Outport  Port=15  VectorParamsAs1DForOutWhenUnconnected=off
  B303_Vang : Outport  Port=16  VectorParamsAs1DForOutWhenUnconnected=off
  B307_Vang : Outport  Port=17  VectorParamsAs1DForOutWhenUnconnected=off
  B310_Vang : Outport  Port=18  VectorParamsAs1DForOutWhenUnconnected=off
  B316_Vang : Outport  Port=19  VectorParamsAs1DForOutWhenUnconnected=off
  B321_Vang : Outport  Port=20  VectorParamsAs1DForOutWhenUnconnected=off
  B323_Vang : Outport  Port=21  VectorParamsAs1DForOutWhenUnconnected=off
  wires:
  Selector20/1 -> B321_Vang/1
  Selector11/1 -> B107_Vang/1
  Selector7/1 -> B123_Vang/1
  Selector6/1 -> B323_Vang/1
  Selector5/1 -> B310_Vang/1
  Selector2/1 -> B302_Vang/1
  Selector3/1 -> B303_Vang/1
  Selector/1 -> B116_Vang/1
  Selector16/1 -> B216_Vang/1
  Selector19/1 -> B316_Vang/1
  Selector10/1 -> B110_Vang/1
  Selector12/1 -> B103_Vang/1
  bus_va/1 -> Selector6/1, Selector20/1, Selector19/1, Selector5/1, Selector4/1, Selector3/1, Selector2/1, Selector18/1, Selector17/1, Selector16/1, Selector15/1, Selector14/1, Selector9/1, Selector8/1, Selector7/1, Selector1/1, Selector/1, Selector10/1, Selector11/1, Selector12/1, Selector13/1
  Selector1/1 -> B121_Vang/1
  Selector4/1 -> B307_Vang/1
  Selector18/1 -> B223_Vang/1
  Selector17/1 -> B221_Vang/1
  Selector13/1 -> B102_Vang/1
  Selector15/1 -> B210_Vang/1
  Selector9/1 -> B203_Vang/1
  Selector14/1 -> B207_Vang/1
  Selector8/1 -> B202_Vang/1

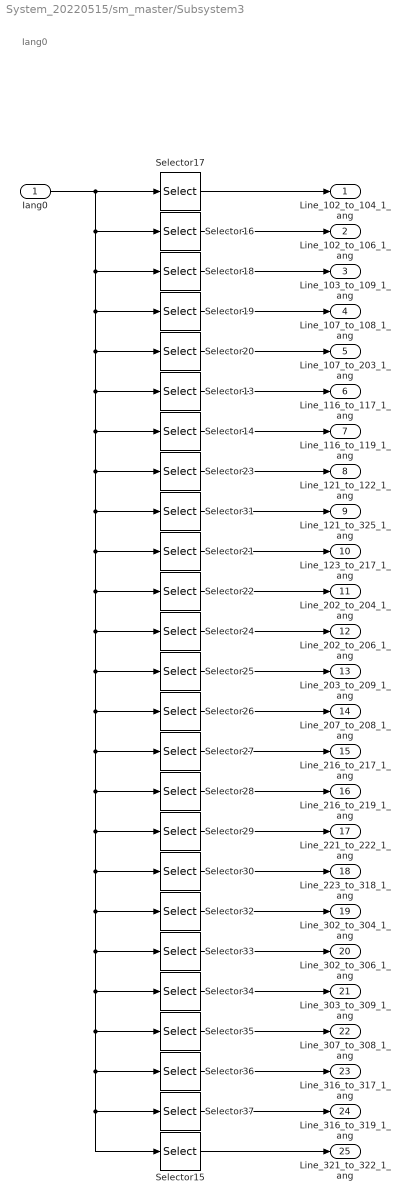
== system System_20220515/sm_master/Subsystem3 ==
  note: Iang0
  Iang0 : Inport
  Selector13 : Selector  InputPortWidth=104  IndexOptions=Index vector (dialog)  Indices=25  OutputSizes=1
  Selector14 : Selector  InputPortWidth=104  IndexOptions=Index vector (dialog)  Indices=26  OutputSizes=1
  Selector15 : Selector  InputPortWidth=104  IndexOptions=Index vector (dialog)  Indices=104  OutputSizes=1
  Selector16 : Selector  InputPortWidth=104  IndexOptions=Index vector (dialog)  Indices=5  OutputSizes=1
  Selector17 : Selector  InputPortWidth=104  IndexOptions=Index vector (dialog)  Indices=4  OutputSizes=1
  Selector18 : Selector  InputPortWidth=104  IndexOptions=Index vector (dialog)  Indices=6  OutputSizes=1
  Selector19 : Selector  InputPortWidth=104  IndexOptions=Index vector (dialog)  Indices=10  OutputSizes=1
  Selector20 : Selector  InputPortWidth=104  IndexOptions=Index vector (dialog)  Indices=11  OutputSizes=1
  Selector21 : Selector  InputPortWidth=104  IndexOptions=Index vector (dialog)  Indices=37  OutputSizes=1
  Selector22 : Selector  InputPortWidth=104  IndexOptions=Index vector (dialog)  Indices=41  OutputSizes=1
  Selector23 : Selector  InputPortWidth=104  IndexOptions=Index vector (dialog)  Indices=35  OutputSizes=1
  Selector24 : Selector  InputPortWidth=104  IndexOptions=Index vector (dialog)  Indices=42  OutputSizes=1
  Selector25 : Selector  InputPortWidth=104  IndexOptions=Index vector (dialog)  Indices=43  OutputSizes=1
  Selector26 : Selector  InputPortWidth=104  IndexOptions=Index vector (dialog)  Indices=47  OutputSizes=1
  Selector27 : Selector  InputPortWidth=104  IndexOptions=Index vector (dialog)  Indices=60  OutputSizes=1
  Selector28 : Selector  InputPortWidth=104  IndexOptions=Index vector (dialog)  Indices=61  OutputSizes=1
  Selector29 : Selector  InputPortWidth=104  IndexOptions=Index vector (dialog)  Indices=70  OutputSizes=1
  Selector30 : Selector  InputPortWidth=104  IndexOptions=Index vector (dialog)  Indices=71  OutputSizes=1
  Selector31 : Selector  InputPortWidth=104  IndexOptions=Index vector (dialog)  Indices=36  OutputSizes=1
  Selector32 : Selector  InputPortWidth=104  IndexOptions=Index vector (dialog)  Indices=75  OutputSizes=1
  Selector33 : Selector  InputPortWidth=104  IndexOptions=Index vector (dialog)  Indices=76  OutputSizes=1
  Selector34 : Selector  InputPortWidth=104  IndexOptions=Index vector (dialog)  Indices=77  OutputSizes=1
  Selector35 : Selector  InputPortWidth=104  IndexOptions=Index vector (dialog)  Indices=81  OutputSizes=1
  Selector36 : Selector  InputPortWidth=104  IndexOptions=Index vector (dialog)  Indices=94  OutputSizes=1
  Selector37 : Selector  InputPortWidth=104  IndexOptions=Index vector (dialog)  Indices=95  OutputSizes=1
  Line_102_to_104_1_ang : Outport  VectorParamsAs1DForOutWhenUnconnected=off
  Line_102_to_106_1_ang : Outport  Port=2  VectorParamsAs1DForOutWhenUnconnected=off
  Line_103_to_109_1_ang : Outport  Port=3  VectorParamsAs1DForOutWhenUnconnected=off
  Line_107_to_108_1_ang : Outport  Port=4  VectorParamsAs1DForOutWhenUnconnected=off
  Line_107_to_203_1_ang : Outport  Port=5  VectorParamsAs1DForOutWhenUnconnected=off
  Line_116_to_117_1_ang : Outport  Port=6  VectorParamsAs1DForOutWhenUnconnected=off
  Line_116_to_119_1_ang : Outport  Port=7  VectorParamsAs1DForOutWhenUnconnected=off
  Line_121_to_122_1_ang : Outport  Port=8  VectorParamsAs1DForOutWhenUnconnected=off
  Line_121_to_325_1_ang : Outport  Port=9  VectorParamsAs1DForOutWhenUnconnected=off
  Line_123_to_217_1_ang : Outport  Port=10  VectorParamsAs1DForOutWhenUnconnected=off
  Line_202_to_204_1_ang : Outport  Port=11  VectorParamsAs1DForOutWhenUnconnected=off
  Line_202_to_206_1_ang : Outport  Port=12  VectorParamsAs1DForOutWhenUnconnected=off
  Line_203_to_209_1_ang : Outport  Port=13  VectorParamsAs1DForOutWhenUnconnected=off
  Line_207_to_208_1_ang : Outport  Port=14  VectorParamsAs1DForOutWhenUnconnected=off
  Line_216_to_217_1_ang : Outport  Port=15  VectorParamsAs1DForOutWhenUnconnected=off
  Line_216_to_219_1_ang : Outport  Port=16  VectorParamsAs1DForOutWhenUnconnected=off
  Line_221_to_222_1_ang : Outport  Port=17  VectorParamsAs1DForOutWhenUnconnected=off
  Line_223_to_318_1_ang : Outport  Port=18  VectorParamsAs1DForOutWhenUnconnected=off
  Line_302_to_304_1_ang : Outport  Port=19  VectorParamsAs1DForOutWhenUnconnected=off
  Line_302_to_306_1_ang : Outport  Port=20  VectorParamsAs1DForOutWhenUnconnected=off
  Line_303_to_309_1_ang : Outport  Port=21  VectorParamsAs1DForOutWhenUnconnected=off
  Line_307_to_308_1_ang : Outport  Port=22  VectorParamsAs1DForOutWhenUnconnected=off
  Line_316_to_317_1_ang : Outport  Port=23  VectorParamsAs1DForOutWhenUnconnected=off
  Line_316_to_319_1_ang : Outport  Port=24  VectorParamsAs1DForOutWhenUnconnected=off
  Line_321_to_322_1_ang : Outport  Port=25  VectorParamsAs1DForOutWhenUnconnected=off
  wires:
  Selector27/1 -> Line_216_to_217_1_ang/1
  Selector29/1 -> Line_221_to_222_1_ang/1
  Selector16/1 -> Line_102_to_106_1_ang/1
  Iang0/1 -> Selector31/1, Selector21/1, Selector22/1, Selector24/1, Selector25/1, Selector26/1, Selector27/1, Selector28/1, Selector30/1, Selector32/1, Selector33/1, Selector34/1, Selector15/1, Selector37/1, Selector36/1, Selector35/1, Selector29/1, Selector23/1, Selector14/1, Selector13/1, Selector20/1, Selector19/1, Selector18/1, Selector16/1, Selector17/1
  Selector32/1 -> Line_302_to_304_1_ang/1
  Selector31/1 -> Line_121_to_325_1_ang/1
  Selector14/1 -> Line_116_to_119_1_ang/1
  Selector35/1 -> Line_307_to_308_1_ang/1
  Selector34/1 -> Line_303_to_309_1_ang/1
  Selector13/1 -> Line_116_to_117_1_ang/1
  Selector28/1 -> Line_216_to_219_1_ang/1
  Selector24/1 -> Line_202_to_206_1_ang/1
  Selector25/1 -> Line_203_to_209_1_ang/1
  Selector18/1 -> Line_103_to_109_1_ang/1
  Selector30/1 -> Line_223_to_318_1_ang/1
  Selector19/1 -> Line_107_to_108_1_ang/1
  Selector22/1 -> Line_202_to_204_1_ang/1
  Selector17/1 -> Line_102_to_104_1_ang/1
  Selector33/1 -> Line_302_to_306_1_ang/1
  Selector15/1 -> Line_321_to_322_1_ang/1
  Selector23/1 -> Line_121_to_122_1_ang/1
  Selector20/1 -> Line_107_to_203_1_ang/1
  Selector36/1 -> Line_316_to_317_1_ang/1
  Selector37/1 -> Line_316_to_319_1_ang/1
  Selector26/1 -> Line_207_to_208_1_ang/1
  Selector21/1 -> Line_123_to_217_1_ang/1
